simulink subsystem "filtro_LP_posicion"  (R2023b)
settings: Solver=VariableStepAuto  StartTime=0.0  StopTime=10.0  RelTol=1e-3
undefined symbols (not defined in the file or in its folder): wn_p, zita
settings Model: Creator=nicol  LastModifiedBy=nicol

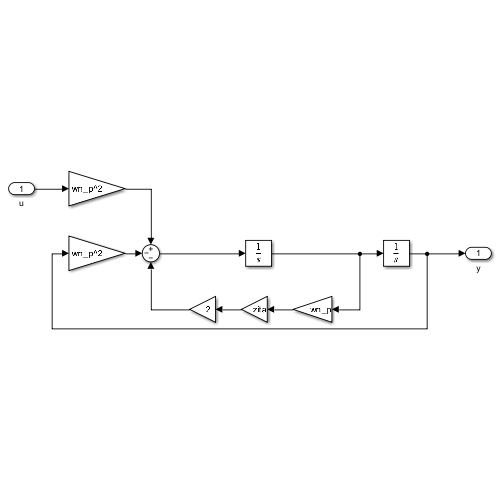
[thumbnail: Simulink's stored preview of the top-level diagram]
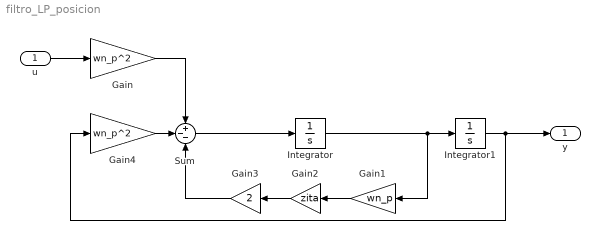
== system filtro_LP_posicion ==
  u : Inport
  Gain : Gain  Gain=wn_p^2
  Gain1 : Gain  Gain=wn_p
  Gain2 : Gain  Gain=zita
  Gain3 : Gain  Gain=2
  Gain4 : Gain  Gain=wn_p^2
  Integrator : Integrator
  Integrator1 : Integrator
  Sum : Sum  Inputs=+--
  y : Outport
  wires:
  Gain2/1 -> Gain3/1
  Gain1/1 -> Gain2/1
  Gain3/1 -> Sum/3
  Sum/1 -> Integrator/1
  Integrator/1 -> Gain1/1, Integrator1/1
  Gain4/1 -> Sum/2
  Gain/1 -> Sum/1
  u/1 -> Gain/1
  Integrator1/1 -> Gain4/1, y/1
